simulink model "eVTOL_PX4_2023b"  (R2024b)
settings: Solver=ode4  StartTime=0  StopTime=inf  FixedStep=0.01  RelTol=1e-3
values from neighbouring files (symbols this model uses):
  aDl =     [initdata.mat]
  aDr =     [initdata.mat]
  aDyn =     [initdata.mat]
  Airport = init_airport('PHNL')    [initdata_HIL_eVTOL.m]
  aLat =     [initdata.mat]
  aLon =     [initdata.mat]
  D = Prop.D    [EOM_dt_MC.m]    (also in EOM_get_alf_dt_de_prop_evtol.m = CD * QS)
  dt0 = X(2)    [EOM_get_alf_dt_de_prop_evtol.m]    (also in initdata.mat = 0.258252593971; initdata_HIL_eVTOL.m = EOM_dt_MC)
  EAS0 = TAS0 / EAS2TAS    [initdata_HIL_eVTOL.m]
  FCS = init_FCS    [initdata_HIL_eVTOL.m]
  General = init_layoutdata    [EOM_dt_MC.m]    (also in build_optimized_CA.m; initdata.mat = ; initdata_HIL_eVTOL.m)
  h0 = Con(1)    [EOM_get_alf_dt_de_prop_evtol.m]    (also in initdata.mat = 450; initdata_HIL_eVTOL.m = 50)
  mass = Con(3)    [EOM_get_alf_dt_de_prop_evtol.m]    (also in initdata.mat = 2255.54; initdata_HIL_eVTOL.m = 7)
  Motor = init_motor_evtol    [EOM_dt_MC.m]    (also in initdata.mat = []; initdata_HIL_eVTOL.m)
  Prop = init_propeller_evtol_new    [EOM_dt_MC.m]    (also in initdata_HIL_eVTOL.m)
  R2D = 180/pi    (= 57.2957795131)    [EOM_get_alf_dt_de_prop_evtol.m]    (also in init_FCS.m; init_aerodata_evtol.m; init_airport.m; initdata.mat)
  SAMPLE_TIME = 0.01    [initdata_HIL_eVTOL.m]
  theta0 = -0.0510981441662    [initdata.mat]
undefined symbols (not defined in the file or in its folder): A1, aDa, aDe, aero, asbhl20env, B1, C1, de0, Earth, Environment, INIT_Data, InitData, Kd, Kp, magnitude, Newton, pProp, Raphson, Tc, WGS84
libraries: simulink_extras x63, vrlib x48, sharedtransform x28, simulink x22, slpidlib x20, sharedutil x20, matrix_library x18, aerolibwindfilters x12, aerolibobsolete x8, aerolibasang x8, aerolibatmos2 x6, aerolibfltsims x6
(part 1 of 17)
settings Model: SimulationMode=accelerator  Creator=Administrator  LastModifiedBy=ZDB
settings SolverCC: EnableFixedStepZeroCrossing=on
settings OptimizationCC: ReuseModelBlockBuffer=off
settings DebuggingCC: UnconnectedInputMsg=warning  UnconnectedOutputMsg=warning  UnconnectedLineMsg=warning
settings ModelReferenceCC: EnableRefExpFcnMdlSchedulingChecks=on
settings RTWCC: GPUComputeCapability=3.5  DLArmComputeVersion=19.05

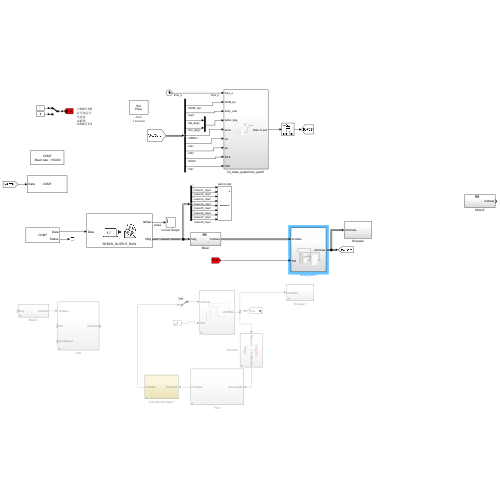
[thumbnail: Simulink's stored preview of the top-level diagram]
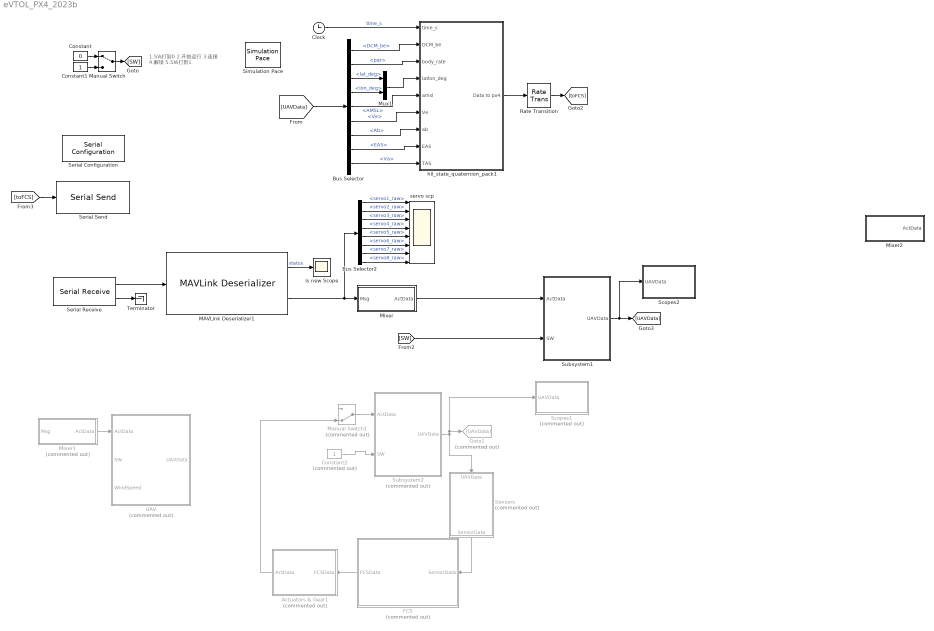
== system eVTOL_PX4_2023b ==
  note: 1.SW打到0
      | 2.开始运行
      | 3.连接
      | 4.解锁
      | 5.SW打到1
  Actuators & Gear1 : Subsystem  Commented=on
  Bus Selector : BusSelector  OutputSignals=DCM_be,pqr,lat_deg,lon_deg,AMSL,Ve,Ab,EAS,Va
  Bus Selector2 : BusSelector  OutputSignals=Payload.servo1_raw,Payload.servo2_raw,Payload.servo3_raw,Payload.servo4_raw,Payload.servo5_raw,Payload.servo6_raw,Payload.servo7_raw,Payload.servo8_raw
  Clock : Clock
  Constant : Constant  Value=0
  Constant1 : Constant
  Constant2 : Constant  Commented=on
  FCS : Subsystem  Commented=on
  Goto1 : Goto  Commented=on  GotoTag=UAVData
  MAVLink Deserializer1 : uavmavlinklib/MAVLink Deserializer  dialectSource=Select from standard MAVLink dialects  dialect=common.xml  dialectCustom=common.xml  version=2  messageType=SERVO_OUTPUT_RAW  inputDataLength=off  SystemIDFilter=off  systemID=1  ComponentIDFilter=off  componentID=1  queueMsg=off  queueMsgSize=50  dropNum=off
  Manual Switch : ManualSwitch
  Manual Switch1 : ManualSwitch  Commented=on  CurrentSetting=0
  Mixer : Subsystem
  Mixer1 : Subsystem  Commented=on
  Mixer2 : Subsystem
  Mux1 : Mux  Inputs=2
  Rate Transition : RateTransition  OutPortSampleTime=0.01
  Scopes1 : Subsystem  Commented=on
  Scopes2 : Subsystem
  Sensors : Subsystem  Commented=on
  Serial Configuration : instrumentseriallib/Serial Configuration  Priority=-200000  PortSel=COM7  Port=COM7  ComPort=COM7  BaudRate=115200  DataBits=8  Parity=none  StopBits=1  ByteOrder=little-endian  FlowControl=none  Timeout=10  SimulateUsing=Interpreted execution  BlockInModel=on  aMode=1
  Serial Receive : instrumentseriallib/Serial Receive  PortSel=COM7  Port=COM7  ComPort=COM7  DataType=uint8  SaveDataType=uint8  ToggleHeader=off  Header=[253 37]  ToggleDataSize=on  DataSize=[49]  ToggleTerminator=off  Terminator=<none>  CustomTerminator=[]  InputFormat=Column major  EnableBlockingMode=off  ActionDataUnavailable=Output last received value  ActionWhenDataUnavailable=Output last received value  CustomValue=0  SampleTime=SAMPLE_TIME  SimulateUsing=Interpreted execution  BlockInModel=on  aMode=1
  Serial Send : instrumentseriallib/Serial Send  Priority=1  PortSel=COM7  Port=COM7  ComPort=COM7  Header=[]  Terminator=<none>  CustomTerminator=[]  EnableBlockingMode=off  SimulateUsing=Interpreted execution  BlockInModel=on  aMode=1
  Simulation Pace : aerolibanimutils/Simulation Pace  SimulationPace=1  SleepMode=Auto  OutputPaceError=off  SampleTime=-1
  Subsystem1 : Subsystem
  Subsystem2 : Subsystem  Commented=on
  Terminator : Terminator
  UAV : Subsystem  Commented=on
  hil_state_quaternion_pack1 : Subsystem
  is new Scope : Scope
  servo scp : Scope  NumInputPorts=8
  wires:
  Actuators & Gear1/1(ActData) -> Manual Switch1/2
  FCS/1(FCSData) -> Actuators & Gear1/1(FCSData)
  Sensors/1(SensorData) -> FCS/1(SensorData)
  Manual Switch/1 -> [SW]
  Bus Selector/5 -> hil_state_quaternion_pack1/5(amsl)  "<AMSL>"
  Bus Selector/4 -> Mux1/2  "<lon_deg>"
  [toFCS] -> Serial Send/1
  Bus Selector/9 -> hil_state_quaternion_pack1/9(TAS)  "<Va>"
  Bus Selector/6 -> hil_state_quaternion_pack1/6(Ve)  "<Ve>"
  Constant1/1 -> Manual Switch/2
  Serial Receive/1 -> MAVLink Deserializer1/1
  MAVLink Deserializer1/1 -> is new Scope/1  "status"
  Constant/1 -> Manual Switch/1
  Bus Selector/8 -> hil_state_quaternion_pack1/8(EAS)  "<EAS>"
  Constant2/1 -> Subsystem2/2(SW)
  Bus Selector/3 -> Mux1/1  "<lat_deg>"
  Bus Selector/1 -> hil_state_quaternion_pack1/2(DCM_be)  "<DCM_be>"
  hil_state_quaternion_pack1/1(Data to px4) -> Rate Transition/1
  Rate Transition/1 -> [toFCS]
  Bus Selector/7 -> hil_state_quaternion_pack1/7(ab)  "<Ab>"
  Mux1/1 -> hil_state_quaternion_pack1/4(latlon_deg)
  Bus Selector/2 -> hil_state_quaternion_pack1/3(body_rate)  "<pqr>"
  [UAVData] -> Bus Selector/1
  Clock/1 -> hil_state_quaternion_pack1/1(time_s)  "time_s"
  Serial Receive/2 -> Terminator/1
  Subsystem2/1(UAVData) -> Goto1/1, Scopes1/1(UAVData), Sensors/1(UAVData)
  Mixer1/1(ActData) -> UAV/1(ActData)
  Manual Switch1/1 -> Subsystem2/1(ActData)
  [SW] -> Subsystem1/2(SW)
  Subsystem1/1(UAVData) -> [UAVData], Scopes2/1(UAVData)
  Bus Selector2/6 -> servo scp/6  "<servo6_raw>"
  Bus Selector2/3 -> servo scp/3  "<servo3_raw>"
  Bus Selector2/4 -> servo scp/4  "<servo4_raw>"
  Bus Selector2/5 -> servo scp/5  "<servo5_raw>"
  MAVLink Deserializer1/2 -> Bus Selector2/1, Mixer/1(Msg)
  Bus Selector2/1 -> servo scp/1  "<servo1_raw>"
  Bus Selector2/2 -> servo scp/2  "<servo2_raw>"
  Bus Selector2/7 -> servo scp/7  "<servo7_raw>"
  Bus Selector2/8 -> servo scp/8  "<servo8_raw>"
  Mixer/1(ActData) -> Subsystem1/1(ActData)

== system eVTOL_PX4_2023b/Actuators & Gear1 ==
  FCSData : Inport
  1-D Lookup Table1 : Lookup_n-D  NumberOfTableDimensions=1  BreakpointsForDimension1=[0, 0.8,1.2,1.57]  Table=[72.43*pi/180,60/57.3,40/57.3, 13*pi/180]  InternalRulePriority=Speed  RndMeth=Simplest
  Bus Creator : BusCreator  Inputs=3
  Bus Creator1 : BusCreator  Inputs=8
  Bus Creator2 : BusCreator  Inputs=2
  Bus Selector : BusSelector  OutputSignals=ACTCMD.dl_cmd,ACTCMD.dt_final,ACTCMD.dr_cmd,ACTCMD.da_cmd,SensorData.Va,FCSCMD.icmd
  Demux : Demux  Outputs=6
  Gain{2,4..11} (9 alike) : Gain
  Max : MinMax  Function=max  Inputs=2
  Mux1 : Mux
  Mux2 : Mux
  Radians to Degrees1 : simulink_extras/Transformations/Radians to Degrees
  Radians to Degrees2 : simulink_extras/Transformations/Radians to Degrees
  Radians to Degrees3 : simulink_extras/Transformations/Radians to Degrees
  Rate Limiter : RateLimiter  FallingSlewLimit=-0.2  SampleTimeMode=inherited
  Saturation1 : Saturate  UpperLimit=25/57.3  LowerLimit=-25/57.3
  Saturation3 : Saturate  UpperLimit=25/57.3  LowerLimit=-25/57.3
  Scope1 : Scope
  Scope2 : Scope
  "[-25,25]" : Saturate  UpperLimit=25/57.3  LowerLimit=-25/57.3
  control output FW : Scope  NumInputPorts=3
  safe i_min : Lookup_n-D  NumberOfTableDimensions=1  BreakpointsForDimension1=[0, 5, 10, 15, 22, 30, 38, 46, 54, 60, 63, 65,80]  Table=[1.22,1.19,1.13,1.05,0.96,0.84,0.7,0.52,0.31,0.14,0.04,0,0]  InternalRulePriority=Speed  RndMeth=Simplest
  ActData : Outport  VectorParamsAs1DForOutWhenUnconnected=off
  tag scope: i=global, theta__b=global
  wires:
  Bus Creator/1 -> Bus Creator2/1  "Act_surface"
  "[-25,25]"/1 -> Radians to Degrees1/1, Bus Creator/2  "dr"
  Saturation3/1 -> Bus Creator/3, Radians to Degrees2/1  "da"
  Saturation1/1 -> Radians to Degrees3/1, Bus Creator/1  "dl"
  Radians to Degrees3/1 -> control output FW/1  "da"
  Radians to Degrees1/1 -> control output FW/2  "de"
  Radians to Degrees2/1 -> control output FW/3  "dr"
  Gain4/1 -> "[-25,25]"/1
  Gain5/1 -> Saturation3/1
  Bus Creator1/1 -> Bus Creator2/2  "Act_T"
  Gain6/1 -> Saturation1/1  "dl"
  FCSData/1 -> Bus Selector/1
  Bus Selector/1 -> Gain6/1  "<dl_cmd>"
  Gain2/1 -> Bus Creator1/1  "dt_1"
  Gain7/1 -> Bus Creator1/2  "dt_2"
  Gain8/1 -> Bus Creator1/3  "dt_3"
  Gain9/1 -> Bus Creator1/4  "dt_4"
  Gain10/1 -> Bus Creator1/5  "dt_5"
  Gain11/1 -> Bus Creator1/6  "dt_6"
  Bus Selector/5 -> safe i_min/1  "<Va>"
  safe i_min/1 -> Max/2
  Max/1 -> Rate Limiter/1  "i"
  1-D Lookup Table1/1 -> [theta__b], Scope2/1  "theta_b"
  Bus Selector/6 -> Max/1  "<icmd>"
  Demux/1 -> Gain2/1
  Demux/2 -> Gain7/1
  Demux/3 -> Gain8/1
  Demux/4 -> Gain9/1
  Demux/5 -> Gain10/1
  Demux/6 -> Gain11/1
  Bus Selector/2 -> Demux/1  "<dt_final>"
  Rate Limiter/1 -> 1-D Lookup Table1/1, Scope1/1, [i]  "i"
  Bus Selector/3 -> Gain4/1  "<dr_cmd>"
  Bus Selector/4 -> Gain5/1  "<da_cmd>"
  Bus Creator2/1 -> ActData/1
  [i] -> Mux1/1  "tilt16"
  [theta__b] -> Mux2/4  "theta_b4"
  [theta__b] -> Mux2/1  "theta_b16"
  [theta__b] -> Mux2/3  "theta_b3"
  [i] -> Mux1/3  "tilt2"
  Mux1/1 -> Bus Creator1/7  "i"
  [i] -> Mux1/4  "tilt5"
  [theta__b] -> Mux2/2  "theta_b25"
  Mux2/1 -> Bus Creator1/8  "theta_b"
  [i] -> Mux1/2  "tilt34"

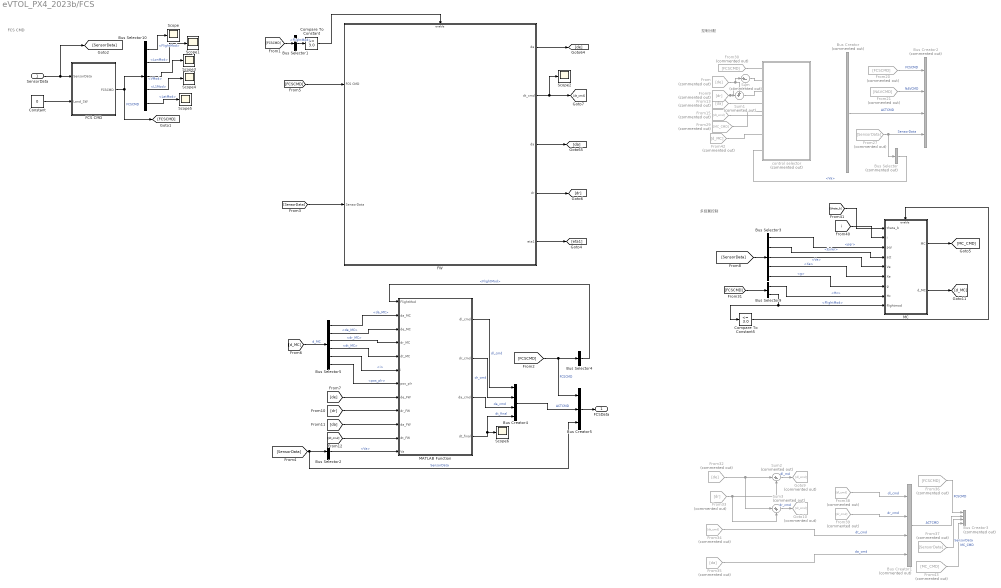
== system eVTOL_PX4_2023b/FCS ==
  note: 控制分配
  note: 多旋翼控制
  note: FCS CMD
  SensorData : Inport
  Bus Creator{,1..3} (4 alike) : BusCreator  Commented=on  Inputs=4
  Bus Creator4 : BusCreator  Inputs=4
  Bus Creator5 : BusCreator  Inputs=3
  Bus Selector : BusSelector  Commented=on  OutputSignals=Va
  Bus Selector1 : BusSelector  OutputSignals=FlightMod
  Bus Selector10 : BusSelector  OutputSignals=FlightMod,LonMod,VMod,L1Mod,LatMod
  Bus Selector2 : BusSelector  OutputSignals=Va
  Bus Selector3 : BusSelector  OutputSignals=pqr,Euler,Ve,Xe,g
  Bus Selector4 : BusSelector  OutputSignals=FlightMod
  Bus Selector5 : BusSelector  OutputSignals=da_MC,de_MC,dr_MC,dt_MC,i,pos_plr
  Bus Selector9 : BusSelector  OutputSignals=Hc,FlightMod
  Compare To Constant : simulink/Logic and Bit Operations/Compare To Constant  relop=>=  const=3.0  OutDataTypeStr=boolean
  Compare To Constant5 : simulink/Logic and Bit Operations/Compare To Constant  relop=<=  const=3.0  OutDataTypeStr=boolean
  Constant : Constant  Value=0
  FCS CMD : Subsystem
  FW : Subsystem
  From : From  Commented=on  GotoTag=de
  From13 : From  Commented=on  GotoTag=da
  From15 : From  Commented=on  GotoTag=dt_cmd
  From20 : From  Commented=on  GotoTag=FCSCMD
      settings: CloseFcn=tagdialog Close
  From21 : From  Commented=on  GotoTag=NAVCMD
      settings: CloseFcn=tagdialog Close
  From27 : From  Commented=on  GotoTag=SensorData
  From29 : From  Commented=on  GotoTag=MC_CMD
  From30 : From  Commented=on  GotoTag=FCSCMD
      settings: CloseFcn=tagdialog Close
  From32 : From  Commented=on  GotoTag=de
  From33 : From  Commented=on  GotoTag=dr
  From34 : From  Commented=on  GotoTag=dt_cmd
  From35 : From  Commented=on  GotoTag=da
  From36 : From  Commented=on  GotoTag=FCSCMD
  From37 : From  Commented=on  GotoTag=SensorData
  From38 : From  Commented=on  GotoTag=dl_cmd
  From39 : From  Commented=on  GotoTag=dr_cmd
  From42 : From  Commented=on  GotoTag=d_MC
  From43 : From  Commented=on  GotoTag=MC_CMD
  From9 : From  Commented=on  GotoTag=dr
  Goto10 : Goto  Commented=on  GotoTag=dr_cmd
  Goto9 : Goto  Commented=on  GotoTag=dl_cmd
  MATLAB Function : MATLAB Function  TreatAsAtomicUnit=on
  MC : Subsystem
  Scope{,1..6} (7 alike) : Scope
  Sum : Sum  Commented=on  Inputs=|+-
  Sum1 : Sum  Commented=on  Inputs=++|
  Sum2 : Sum  Commented=on  Inputs=|+-
  Sum3 : Sum  Commented=on  Inputs=|++
  control selector : Subsystem  Commented=on
  FCSData : Outport  VectorParamsAs1DForOutWhenUnconnected=off
  wires:
  Bus Creator/1 -> Bus Creator2/3  "ACTCMD"
  SensorData/1 -> FCS CMD/1(SensorData), [SensorData]
  FCS CMD/1(FCSCMD) -> Bus Selector10/1, [FCSCMD]  "FCSCMD"
  From20/1 -> Bus Creator2/1  "FCSCMD"
  From21/1 -> Bus Creator2/2  "NAVCMD"
  From30/1 -> ?
  [SensorData] -> Bus Selector3/1
  Bus Selector3/1 -> MC/3(pqr)  "<pqr>"
  Bus Selector3/2 -> MC/4(att)  "<Euler>"
  Bus Selector3/3 -> MC/5(Ve)  "<Ve>"
  Bus Selector3/4 -> MC/6(Xe)  "<Xe>"
  Constant/1 -> FCS CMD/2(Land_SW)
  Bus Selector3/5 -> MC/7(g)  "<g>"
  From/1 -> Sum1/1, Sum/1
  From9/1 -> Sum/2, Sum1/2
  Sum/1 -> ?
  Sum1/1 -> ?
  From13/1 -> ?
  From15/1 -> ?
  From27/1 -> Bus Selector/1, Bus Creator2/4  "SensorData"
  From29/1 -> ?
  Bus Selector/1 -> ?  "<Va>"
  [FCSCMD] -> Bus Selector9/1
  Bus Selector9/1 -> MC/8(Hc)  "<Hc>"
  Bus Selector10/1 -> Scope/1  "<FlightMod>"
  Bus Selector10/2 -> Scope1/1  "<LonMod>"
  Bus Selector10/3 -> Scope3/1  "<VMod>"
  Bus Selector10/4 -> Scope4/1  "<L1Mod>"
  Bus Selector10/5 -> Scope5/1  "<LatMod>"
  From33/1 -> Sum3/2, Sum2/2
  From32/1 -> Sum3/1, Sum2/1
  From34/1 -> Bus Creator1/3  "dt_cmd"
  From35/1 -> Bus Creator1/4  "da_cmd"
  Bus Creator1/1 -> Bus Creator3/2  "ACTCMD"
  From36/1 -> Bus Creator3/1  "FCSCMD"
  From37/1 -> Bus Creator3/3  "SensorData"
  Sum2/1 -> Goto9/1  "dl_md"
  Sum3/1 -> Goto10/1  "dr_cmd"
  From39/1 -> Bus Creator1/2  "dr_cmd"
  From38/1 -> Bus Creator1/1  "dl_cmd"
  Bus Selector9/2 -> Compare To Constant5/1, MC/9(flightmod)  "<FlightMod>"
  [i] -> MC/2(i)
  [theta_b] -> MC/1(theta_b)
  From42/1 -> ?
  ? -> Bus Creator/1  "dl_cmd"
  ? -> Bus Creator/2  "dr_cmd"
  ? -> Bus Creator/3  "da_cmd"
  ? -> Bus Creator/4  "dt_cmd"
  From43/1 -> Bus Creator3/4  "MC_CMD"
  FW/1(de) -> [de]
  [FCSCMD] -> FW/1(FCS CMD)
  [SensorData] -> FW/2(SensorData)
  FW/5(eta1) -> [eta1]
  FW/4(dr) -> [dr]
  FW/3(da) -> [da]
  FW/2(dt_cmd) -> Scope2/1, [dt_cmd]
  [FCSCMD] -> Bus Selector1/1
  Bus Selector1/1 -> Compare To Constant/1  "<FlightMod>"
  Compare To Constant/1 -> FW/Enable
  MATLAB Function/1(dl_cmd) -> Bus Creator4/1  "dl_cmd"
  MATLAB Function/2(dr_cmd) -> Bus Creator4/2  "dr_cmd"
  MATLAB Function/3(da_cmd) -> Bus Creator4/3  "da_cmd"
  MATLAB Function/4(dt_final) -> Scope6/1, Bus Creator4/4  "dt_final"
  Bus Creator4/1 -> Bus Creator5/2  "ACTCMD"
  [SensorData] -> Bus Creator5/3, Bus Selector2/1  "SensorData"
  Bus Selector2/1 -> MATLAB Function/12(Va)  "<Va>"
  [FCSCMD] -> Bus Selector4/1, Bus Creator5/1  "FCSCMD"
  Bus Creator5/1 -> FCSData/1
  Bus Selector4/1 -> MATLAB Function/1(FlightMod)  "<FlightMod>"
  [d_MC] -> Bus Selector5/1  "d_MC"
  Bus Selector5/6 -> MATLAB Function/7(pos_plr)  "<pos_plr>"
  Bus Selector5/1 -> MATLAB Function/2(da_MC)  "<da_MC>"
  Bus Selector5/2 -> MATLAB Function/3(de_MC)  "<de_MC>"
  Bus Selector5/3 -> MATLAB Function/4(dr_MC)  "<dr_MC>"
  Bus Selector5/4 -> MATLAB Function/5(dt_MC)  "<dt_MC>"
  Bus Selector5/5 -> MATLAB Function/6(i)  "<i>"
  [de] -> MATLAB Function/8(de_FW)
  [dr] -> MATLAB Function/9(dr_FW)
  [da] -> MATLAB Function/10(da_FW)
  [dt_cmd] -> MATLAB Function/11(dt_FW)
  MC/1(MC) -> [MC_CMD]
  MC/2(d_MC) -> [d_MC]
  Compare To Constant5/1 -> MC/Enable

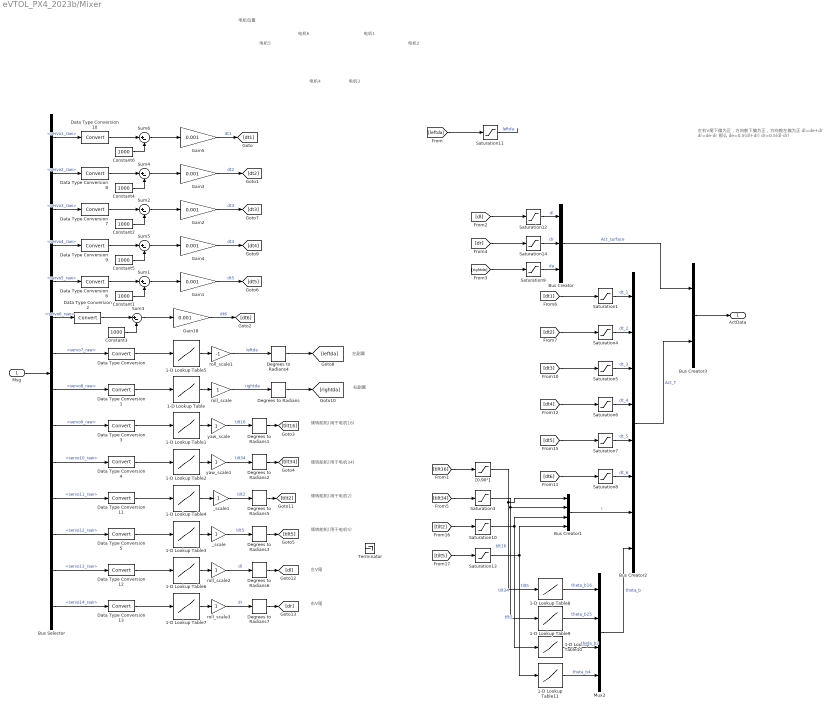
== system eVTOL_PX4_2023b/Mixer ==
  note: 电机1
  note: 电机位置
  note: 左副翼
  note: 左右V尾下偏为正，方向舵下偏为正，方向舵左偏为正
      | dl=de+dr
      | dr=de-dr
      | 那么
      | de=0.5(dl+dr)
      | dr=0.5(dl-dr)
  note: 右副翼
  note: 倾转舵机(用于电机16)
  note: 左V尾
  note: 右V尾
  note: 倾转舵机(用于电机34)
  note: 倾转舵机(用于电机2)
  note: 倾转舵机(用于电机5)
  note: 电机2
  note: 电机3
  note: 电机4
  note: 电机5
  note: 电机6
  Msg : Inport
  1-D Lookup Table{,5..7} (4 alike) : Lookup_n-D  NumberOfTableDimensions=1  BreakpointsForDimension1=[1000, 1500, 2000]  Table=[-30, 0, 30]  InternalRulePriority=Speed  RndMeth=Simplest
  1-D Lookup Table{1..4} (4 alike) : Lookup_n-D  NumberOfTableDimensions=1  BreakpointsForDimension1=[1000, 1500, 2000]  Table=[90, 45, 0]  InternalRulePriority=Speed  RndMeth=Simplest
  1-D Lookup Table{8..11} (4 alike) : Lookup_n-D  NumberOfTableDimensions=1  BreakpointsForDimension1=[0, 0.8,1.2,1.57]  Table=[72.43*pi/180,60/57.3,40/57.3, 13*pi/180]  InternalRulePriority=Speed  RndMeth=Simplest
  Bus Creator : BusCreator  Inputs=3
  Bus Creator1 : BusCreator  Inputs=4
  Bus Creator2 : BusCreator  Inputs=8
  Bus Creator3 : BusCreator  Inputs=2
  Bus Selector : BusSelector  OutputSignals=Payload.servo1_raw,Payload.servo2_raw,Payload.servo3_raw,Payload.servo4_raw,Payload.servo5_raw,Payload.servo6_raw,Payload.servo7_raw,Payload.servo8_raw,Payload.servo9_raw,Payload.servo10_raw,Payload.servo11_raw,Payload.servo12_raw,Payload.servo13_raw,Payload.servo14_raw
  Constant{1..6} (6 alike) : Constant  Value=1000
  Data Type Conversion{,1..13} (14 alike) : DataTypeConversion  SaturateOnIntegerOverflow=off  RndMeth=Floor
  Degrees to Radians{,1..7} (8 alike) : simulink_extras/Transformations/Degrees to Radians
  Gain{1..5,18} (6 alike) : Gain  Gain=0.001
  Mux2 : Mux
  Saturation{1,4..8} (6 alike) : Saturate  UpperLimit=1  LowerLimit=0
  Saturation10 : Saturate  UpperLimit=90/57.3  LowerLimit=0
  Saturation{9,11..12,14} (4 alike) : Saturate  UpperLimit=25/57.3  LowerLimit=-25/57.3
  Saturation13 : Saturate  UpperLimit=90/57.3  LowerLimit=0
  Saturation3 : Saturate  UpperLimit=90/57.3  LowerLimit=0
  Sum{1..6} (6 alike) : Sum  Inputs=|+-
  Terminator : Terminator
  "[0,90°]" : Saturate  UpperLimit=90/57.3  LowerLimit=0
  _scale : Gain
  _scale1 : Gain
  roll_scale : Gain
  roll_scale1 : Gain  Gain=-1
  roll_scale2 : Gain
  roll_scale3 : Gain
  yaw_scale : Gain
  yaw_scale1 : Gain
  ActData : Outport  VectorParamsAs1DForOutWhenUnconnected=off
  wires:
  Bus Selector/6 -> Data Type Conversion2/1  "<servo6_raw>"
  Bus Selector/7 -> Data Type Conversion/1  "<servo7_raw>"
  Bus Selector/8 -> Data Type Conversion1/1  "<servo8_raw>"
  Constant3/1 -> Sum3/2
  Sum3/1 -> Gain18/1
  Degrees to Radians4/1 -> [leftda]
  Degrees to Radians/1 -> [rightda]
  1-D Lookup Table1/1 -> yaw_scale/1
  [leftda] -> Saturation11/1
  Saturation11/1 -> ?  "leftda"
  [dl] -> Saturation12/1
  Saturation12/1 -> Bus Creator/1  "dl"
  "[0,90°]"/1 -> 1-D Lookup Table8/1, Bus Creator1/1  "tilt16"
  Saturation3/1 -> 1-D Lookup Table9/1, Bus Creator1/2  "tilt34"
  1-D Lookup Table3/1 -> _scale/1
  1-D Lookup Table2/1 -> yaw_scale1/1
  Gain18/1 -> [dt6]  "dt6"
  Bus Selector/9 -> Data Type Conversion3/1  "<servo9_raw>"
  Bus Selector/10 -> Data Type Conversion4/1  "<servo10_raw>"
  Degrees to Radians1/1 -> [tilt16]
  Degrees to Radians2/1 -> [tilt34]
  Degrees to Radians3/1 -> [tilt5]
  _scale/1 -> Degrees to Radians3/1  "tilt5"
  yaw_scale/1 -> Degrees to Radians1/1  "tilt16"
  yaw_scale1/1 -> Degrees to Radians2/1  "tilt34"
  Data Type Conversion/1 -> 1-D Lookup Table5/1
  Data Type Conversion1/1 -> 1-D Lookup Table/1
  Data Type Conversion3/1 -> 1-D Lookup Table1/1
  Data Type Conversion4/1 -> 1-D Lookup Table2/1
  Data Type Conversion5/1 -> 1-D Lookup Table3/1
  roll_scale/1 -> Degrees to Radians/1  "rightda"
  1-D Lookup Table/1 -> roll_scale/1
  [dr] -> Saturation14/1
  [tilt16] -> "[0,90°]"/1
  [tilt34] -> Saturation3/1
  1-D Lookup Table5/1 -> roll_scale1/1
  roll_scale1/1 -> Degrees to Radians4/1  "leftda"
  Data Type Conversion2/1 -> Sum3/1
  Bus Selector/5 -> Data Type Conversion6/1  "<servo5_raw>"
  Constant1/1 -> Sum1/2
  Data Type Conversion6/1 -> Sum1/1
  Sum1/1 -> Gain1/1
  Gain1/1 -> [dt5]  "dt5"
  Bus Selector/4 -> Data Type Conversion9/1  "<servo4_raw>"
  Constant5/1 -> Sum5/2
  Data Type Conversion9/1 -> Sum5/1
  Sum5/1 -> Gain4/1
  Gain4/1 -> [dt4]  "dt4"
  Bus Selector/3 -> Data Type Conversion7/1  "<servo3_raw>"
  Constant2/1 -> Sum2/2
  Data Type Conversion7/1 -> Sum2/1
  Sum2/1 -> Gain2/1
  Gain2/1 -> [dt3]  "dt3"
  Bus Selector/2 -> Data Type Conversion8/1  "<servo2_raw>"
  Constant4/1 -> Sum4/2
  Data Type Conversion8/1 -> Sum4/1
  Sum4/1 -> Gain3/1
  Gain3/1 -> [dt2]  "dt2"
  Bus Selector/1 -> Data Type Conversion10/1  "<servo1_raw>"
  Constant6/1 -> Sum6/2
  Data Type Conversion10/1 -> Sum6/1
  Sum6/1 -> Gain5/1
  Gain5/1 -> [dt1]  "dt1"
  Data Type Conversion11/1 -> 1-D Lookup Table4/1
  Degrees to Radians5/1 -> [tilt2]
  _scale1/1 -> Degrees to Radians5/1  "tilt2"
  Bus Selector/11 -> Data Type Conversion11/1  "<servo11_raw>"
  1-D Lookup Table4/1 -> _scale1/1
  Data Type Conversion12/1 -> 1-D Lookup Table6/1
  Degrees to Radians6/1 -> [dl]
  roll_scale2/1 -> Degrees to Radians6/1  "dl"
  Bus Selector/13 -> Data Type Conversion12/1  "<servo13_raw>"
  1-D Lookup Table6/1 -> roll_scale2/1
  Data Type Conversion13/1 -> 1-D Lookup Table7/1
  Degrees to Radians7/1 -> [dr]
  roll_scale3/1 -> Degrees to Radians7/1  "dr"
  Bus Selector/14 -> Data Type Conversion13/1  "<servo14_raw>"
  1-D Lookup Table7/1 -> roll_scale3/1
  Bus Selector/12 -> Data Type Conversion5/1  "<servo12_raw>"
  [dt1] -> Saturation1/1
  Saturation1/1 -> Bus Creator2/1  "dt_1"
  [dt2] -> Saturation4/1
  Saturation4/1 -> Bus Creator2/2  "dt_2"
  [dt3] -> Saturation5/1
  Saturation5/1 -> Bus Creator2/3  "dt_3"
  Saturation7/1 -> Bus Creator2/5  "dt_5"
  Saturation6/1 -> Bus Creator2/4  "dt_4"
  [dt4] -> Saturation6/1
  [dt6] -> Saturation8/1
  Saturation8/1 -> Bus Creator2/6  "dt_6"
  [dt5] -> Saturation7/1
  [rightda] -> Saturation9/1
  Saturation9/1 -> Bus Creator/3  "da"
  [tilt2] -> Saturation10/1
  Saturation10/1 -> Bus Creator1/3, 1-D Lookup Table10/1  "tilt2"
  [tilt5] -> Saturation13/1
  Saturation13/1 -> Bus Creator1/4, 1-D Lookup Table11/1  "tilt5"
  Bus Creator3/1 -> ActData/1
  Bus Creator2/1 -> Bus Creator3/2  "Act_T"
  Bus Creator/1 -> Bus Creator3/1  "Act_surface"
  Saturation14/1 -> Bus Creator/2  "dr"
  Bus Creator1/1 -> Bus Creator2/7  "i"
  1-D Lookup Table8/1 -> Mux2/1  "theta_b16"
  1-D Lookup Table9/1 -> Mux2/2  "theta_b25"
  1-D Lookup Table10/1 -> Mux2/3  "theta_b3"
  1-D Lookup Table11/1 -> Mux2/4  "theta_b4"
  Mux2/1 -> Bus Creator2/8  "theta_b"
  Msg/1 -> Bus Selector/1
  ? -> ?  "y轴"
  ? -> ?  "x轴"

== system eVTOL_PX4_2023b/Mixer1 ==
  Msg : Inport
  1-D Lookup Table{,1..3,5} (5 alike) : Lookup_n-D  NumberOfTableDimensions=1  BreakpointsForDimension1=[1000, 1500, 2000]  Table=[-20, 0, 20]  InternalRulePriority=Speed  RndMeth=Simplest
  Bus Creator1 : BusCreator  Inputs=6
  Bus Selector : BusSelector  OutputSignals=Payload.servo1_raw,Payload.servo2_raw,Payload.servo3_raw,Payload.servo4_raw,Payload.servo5_raw,Payload.servo6_raw
  Constant3 : Constant  Value=1000
  Data Type Conversion{,1..5} (6 alike) : DataTypeConversion  SaturateOnIntegerOverflow=off  RndMeth=Floor
  Degrees to Radians{,1..4} (5 alike) : simulink_extras/Transformations/Degrees to Radians
  Gain18 : Gain  Gain=0.001
  Radians to Degrees : simulink_extras/Transformations/Radians to Degrees
  Radians to Degrees4 : simulink_extras/Transformations/Radians to Degrees
  Radians to Degrees5 : simulink_extras/Transformations/Radians to Degrees
  Saturation11 : Saturate  UpperLimit=1  LowerLimit=-1
  Saturation12 : Saturate  UpperLimit=1  LowerLimit=-1
  Saturation13 : Saturate  UpperLimit=1  LowerLimit=0
  Saturation14 : Saturate  UpperLimit=25/57.3  LowerLimit=-25/57.3
  Saturation2 : Saturate  UpperLimit=25/57.3  LowerLimit=-25/57.3
  Saturation3 : Saturate  UpperLimit=25/57.3  LowerLimit=-25/57.3
  Sum3 : Sum  Inputs=|+-
  da Scope : Scope
  de Scope : Scope
  dr Scope : Scope
  dt Scope : Scope
  pitch_scale : Gain  Gain=-1
  pitch_scale1 : Gain  Gain=-1
  roll_scale : Gain
  yaw_scale : Gain  Gain=-1
  yaw_scale1 : Gain
  ActData : Outport
  wires:
  Data Type Conversion2/1 -> Sum3/1
  pitch_scale1/1 -> Degrees to Radians4/1
  1-D Lookup Table5/1 -> pitch_scale1/1
  [dt6] -> Saturation3/1
  [dt5] -> Saturation2/1
  [dt4] -> Saturation14/1
  1-D Lookup Table/1 -> pitch_scale/1
  pitch_scale/1 -> Degrees to Radians/1
  Data Type Conversion5/1 -> 1-D Lookup Table3/1
  Data Type Conversion4/1 -> 1-D Lookup Table2/1
  Data Type Conversion3/1 -> 1-D Lookup Table1/1
  Data Type Conversion1/1 -> 1-D Lookup Table/1
  Data Type Conversion/1 -> 1-D Lookup Table5/1
  yaw_scale1/1 -> Degrees to Radians2/1
  yaw_scale/1 -> Degrees to Radians1/1
  roll_scale/1 -> Degrees to Radians3/1
  Radians to Degrees5/1 -> da Scope/1  "da"
  [dt1] -> Radians to Degrees5/1
  [dt4] -> Radians to Degrees4/1
  Radians to Degrees4/1 -> dr Scope/1  "dr"
  Degrees to Radians3/1 -> [dt6]
  Degrees to Radians2/1 -> [dt5]
  Degrees to Radians1/1 -> [dt4]
  Bus Selector/6 -> Data Type Conversion5/1  "<servo6_raw>"
  Bus Selector/5 -> Data Type Conversion4/1  "<servo5_raw>"
  Bus Selector/4 -> Data Type Conversion3/1  "<servo4_raw>"
  [dt3] -> dt Scope/1  "throttle"
  Radians to Degrees/1 -> de Scope/1  "de"
  Gain18/1 -> [dt3]
  [dt2] -> Radians to Degrees/1
  1-D Lookup Table2/1 -> yaw_scale1/1
  1-D Lookup Table3/1 -> roll_scale/1
  Saturation3/1 -> Bus Creator1/6  "wheel"
  Saturation2/1 -> Bus Creator1/5  "flap"
  Saturation14/1 -> Bus Creator1/4  "dr"
  Saturation13/1 -> Bus Creator1/3  "dt"
  [dt3] -> Saturation13/1
  Saturation12/1 -> Bus Creator1/2  "de"
  [dt2] -> Saturation12/1
  Saturation11/1 -> Bus Creator1/1  "da"
  [dt1] -> Saturation11/1
  1-D Lookup Table1/1 -> yaw_scale/1
  Degrees to Radians/1 -> [dt2]  "dt1"
  Degrees to Radians4/1 -> [dt1]  "dt1"
  Bus Creator1/1 -> ActData/1
  Sum3/1 -> Gain18/1
  Constant3/1 -> Sum3/2
  Bus Selector/2 -> Data Type Conversion1/1  "<servo2_raw>"
  Bus Selector/1 -> Data Type Conversion/1  "<servo1_raw>"
  Bus Selector/3 -> Data Type Conversion2/1  "<servo3_raw>"
  Msg/1 -> Bus Selector/1

== system eVTOL_PX4_2023b/Mixer2 ==
  note: 电机1
  note: 电机位置
  note: 左右V尾下偏为正，方向舵下偏为正，方向舵左偏为正
      | dl=de+dr
      | dr=de-dr
      | 那么
      | de=0.5(dl+dr)
      | dr=0.5(dl-dr)
  note: 电机2
  note: 电机3
  note: 电机4
  note: 电机5
  note: 电机6
  0.63 : Step  Time=10  After=0.63  SampleTime=0
  0.67 : Step  Time=10  After=0.67  SampleTime=0
  0.7 : Step  Time=10  After=0.7  SampleTime=0
  1-D Lookup Table{8..11} (4 alike) : Lookup_n-D  NumberOfTableDimensions=1  BreakpointsForDimension1=[0, 0.8,1.2,1.57]  Table=[72.43*pi/180,60/57.3,40/57.3, 13*pi/180]  InternalRulePriority=Speed  RndMeth=Simplest
  Bus Creator : BusCreator  Inputs=3
  Bus Creator2 : BusCreator  Inputs=8
  Bus Creator3 : BusCreator  Inputs=2
  Constant13 : Constant  Value=0
  Constant7 : Constant  Value=1.57
  Mux1 : Mux
  Mux2 : Mux
  Saturation{1,4..8} (6 alike) : Saturate  UpperLimit=1  LowerLimit=0
  Saturation10 : Saturate  UpperLimit=90/57.3  LowerLimit=0
  Saturation12 : Saturate  UpperLimit=25/57.3  LowerLimit=-25/57.3
  Saturation13 : Saturate  UpperLimit=90/57.3  LowerLimit=0
  Saturation14 : Saturate  UpperLimit=25/57.3  LowerLimit=-25/57.3
  Saturation3 : Saturate  UpperLimit=90/57.3  LowerLimit=0
  Saturation9 : Saturate  UpperLimit=25/57.3  LowerLimit=-25/57.3
  "[0,90°]" : Saturate  UpperLimit=90/57.3  LowerLimit=0
  ActData : Outport  VectorParamsAs1DForOutWhenUnconnected=off
  wires:
  Saturation12/1 -> Bus Creator/1  "dl"
  "[0,90°]"/1 -> 1-D Lookup Table8/1, Mux1/1  "tilt16"
  Saturation3/1 -> 1-D Lookup Table9/1, Mux1/2  "tilt34"
  Constant7/1 -> Saturation10/1, Saturation3/1, "[0,90°]"/1, Saturation13/1
  Saturation1/1 -> Bus Creator2/1  "dt_1"
  Saturation4/1 -> Bus Creator2/2  "dt_2"
  Saturation5/1 -> Bus Creator2/3  "dt_3"
  Saturation7/1 -> Bus Creator2/5  "dt_5"
  Saturation6/1 -> Bus Creator2/4  "dt_4"
  Saturation8/1 -> Bus Creator2/6  "dt_6"
  Constant13/1 -> Saturation9/1, Saturation14/1, Saturation12/1
  Saturation9/1 -> Bus Creator/3  "da"
  Saturation10/1 -> 1-D Lookup Table10/1, Mux1/3  "tilt2"
  Saturation13/1 -> 1-D Lookup Table11/1, Mux1/4  "tilt5"
  Bus Creator3/1 -> ActData/1
  Bus Creator2/1 -> Bus Creator3/2  "Act_T"
  Bus Creator/1 -> Bus Creator3/1  "Act_surface"
  Saturation14/1 -> Bus Creator/2  "dr"
  Mux1/1 -> Bus Creator2/7  "i"
  1-D Lookup Table8/1 -> Mux2/1  "theta_b16"
  1-D Lookup Table9/1 -> Mux2/2  "theta_b25"
  1-D Lookup Table10/1 -> Mux2/3  "theta_b3"
  1-D Lookup Table11/1 -> Mux2/4  "theta_b4"
  Mux2/1 -> Bus Creator2/8  "theta_b"
  ? -> ?  "y轴"
  ? -> ?  "x轴"
  0.7/1 -> Saturation8/1, Saturation1/1
  0.67/1 -> Saturation7/1, Saturation4/1
  0.63/1 -> Saturation6/1, Saturation5/1

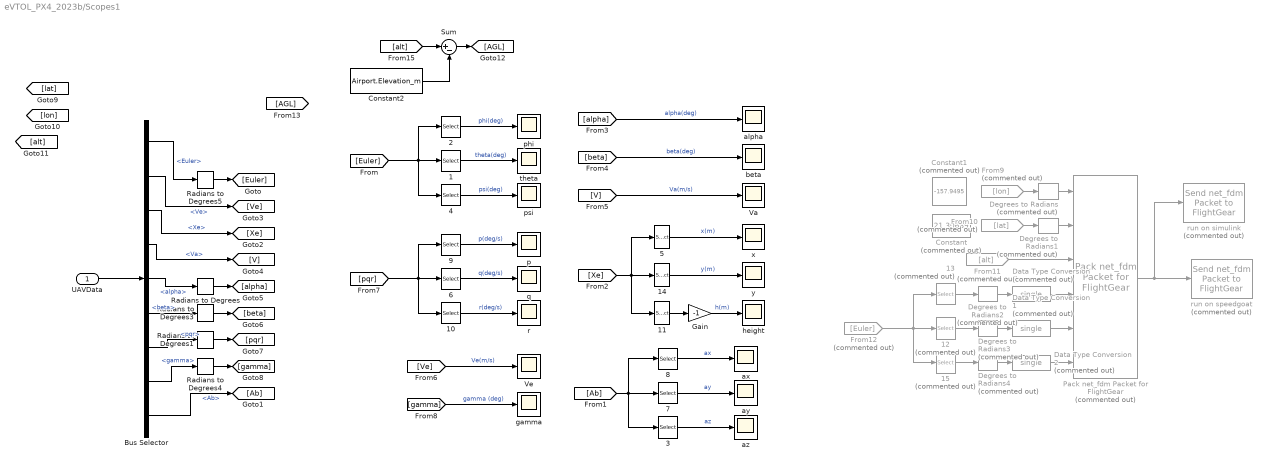
== system eVTOL_PX4_2023b/Scopes1 ==
  UAVData : Inport
  {1,6..7,14} (4 alike) : Selector  InputPortWidth=3  IndexOptions=Index vector (dialog)  Indices=2  OutputSizes=1
  {3..4,10..11} (4 alike) : Selector  InputPortWidth=3  IndexOptions=Index vector (dialog)  Indices=3  OutputSizes=1
  12 : Selector  Commented=on  InputPortWidth=3  IndexOptions=Index vector (dialog)  Indices=2  OutputSizes=1
  13 : Selector  Commented=on  InputPortWidth=3  IndexOptions=Index vector (dialog)  Indices=1  OutputSizes=1
  15 : Selector  Commented=on  InputPortWidth=3  IndexOptions=Index vector (dialog)  Indices=3  OutputSizes=1
  {2,5,8..9} (4 alike) : Selector  InputPortWidth=3  IndexOptions=Index vector (dialog)  Indices=1  OutputSizes=1
  Bus Selector : BusSelector  OutputSignals=Euler,Ve,Xe,Va,alpha,beta,pqr,gamma,Ab
  Constant : Constant  Commented=on  Value=21.30689
  Constant1 : Constant  Commented=on  Value=-157.9495
  Constant2 : Constant  Value=Airport.Elevation_m
  Data Type Conversion : DataTypeConversion  Commented=on  OutDataTypeStr=single  SaturateOnIntegerOverflow=off  RndMeth=Floor
  Data Type Conversion1 : DataTypeConversion  Commented=on  OutDataTypeStr=single  SaturateOnIntegerOverflow=off  RndMeth=Floor
  Data Type Conversion2 : DataTypeConversion  Commented=on  OutDataTypeStr=single  SaturateOnIntegerOverflow=off  RndMeth=Floor
  Degrees to Radians{,1..4} (5 alike) : simulink_extras/Transformations/Degrees to Radians  Commented=on
  From10 : From  Commented=on  GotoTag=lat
  From11 : From  Commented=on  GotoTag=alt
  From12 : From  Commented=on  GotoTag=Euler
  From9 : From  Commented=on  GotoTag=lon
  Gain : Gain  Gain=-1
  Pack net_fdm Packet for FlightGear : aerolibfltsims/Pack net_fdm Packet for FlightGear  Commented=on  FlightGearVersion=v2019.1  ShowPositionAttitudeInputs=on  ShowVelocityAccelerationInputs=off  ShowControlSurfacePositionInputs=off  ShowEngineFuelInputs=off  ShowLandingGearInputs=off  ShowEnvironmentInputs=off  SampleTime=-1  packetVersion=24
  Radians to Degrees{,1,3..5} (5 alike) : simulink_extras/Transformations/Radians to Degrees
  Sum : Sum  Inputs=|+-
  Va : Scope
  Ve : Scope
  alpha : Scope
  ax : Scope
  ay : Scope
  az : Scope
  beta : Scope
  gamma : Scope
  height : Scope
  p : Scope
  phi : Scope
  psi : Scope
  q : Scope
  r : Scope
  run on simulink : aerolibfltsims/Send net_fdm Packet to FlightGear  Commented=on  DestinationIpAddress=127.0.0.1  DestinationPort=5502  LocalIpPort=-1  varLen=off  SampleTime=0.01
  run on speedgoat : aerolibfltsims/Send net_fdm Packet to FlightGear  Commented=on  DestinationIpAddress=192.168.7.2  DestinationPort=5502  LocalIpPort=-1  varLen=off  SampleTime=-1
  theta : Scope
  x : Scope
  y : Scope
  wires:
  Radians to Degrees5/1 -> [Euler]
  UAVData/1 -> Bus Selector/1
  1/1 -> theta/1  "theta(deg)"
  Bus Selector/3 -> [Xe]  "<Xe>"
  2/1 -> phi/1  "phi(deg)"
  4/1 -> psi/1  "psi(deg)"
  Bus Selector/5 -> Radians to Degrees/1  "<alpha>"
  [Euler] -> 1/1, 2/1, 4/1
  Bus Selector/1 -> Radians to Degrees5/1  "<Euler>"
  [Xe] -> 5/1, 14/1, 11/1
  Bus Selector/2 -> [Ve]  "<Ve>"
  Bus Selector/4 -> [V]  "<Va>"
  Radians to Degrees/1 -> [alpha]
  Bus Selector/6 -> Radians to Degrees3/1  "<beta>"
  Radians to Degrees3/1 -> [beta]
  [beta] -> beta/1  "beta(deg)"
  [alpha] -> alpha/1  "alpha(deg)"
  [Ve] -> Ve/1  "Ve(m/s)"
  Bus Selector/7 -> Radians to Degrees1/1  "<pqr>"
  6/1 -> q/1  "q(deg/s)"
  9/1 -> p/1  "p(deg/s)"
  10/1 -> r/1  "r(deg/s)"
  [pqr] -> 10/1, 9/1, 6/1
  Radians to Degrees1/1 -> [pqr]
  11/1 -> Gain/1
  Gain/1 -> height/1  "h(m)"
  5/1 -> x/1  "x(m)"
  Bus Selector/8 -> Radians to Degrees4/1  "<gamma>"
  Radians to Degrees4/1 -> [gamma]
  [gamma] -> gamma/1  "gamma (deg)"
  14/1 -> y/1  "y(m)"
  [V] -> Va/1  "Va(m/s)"
  Bus Selector/9 -> [Ab]  "<Ab>"
  [Ab] -> 8/1, 7/1, 3/1
  3/1 -> az/1  "az"
  8/1 -> ax/1  "ax"
  7/1 -> ay/1  "ay"
  ? -> [lat]  "<lat_deg>"
  ? -> [lon]  "<lon_deg>"
  ? -> [alt]  "<AMSL>"
  Pack net_fdm Packet for FlightGear/1 -> run on simulink/1, run on speedgoat/1
  Degrees to Radians1/1 -> Pack net_fdm Packet for FlightGear/2
  Data Type Conversion/1 -> Pack net_fdm Packet for FlightGear/4
  Degrees to Radians/1 -> Pack net_fdm Packet for FlightGear/1
  12/1 -> Degrees to Radians3/1
  Data Type Conversion1/1 -> Pack net_fdm Packet for FlightGear/5
  13/1 -> Degrees to Radians2/1
  15/1 -> Degrees to Radians4/1
  Data Type Conversion2/1 -> Pack net_fdm Packet for FlightGear/6
  From11/1 -> Pack net_fdm Packet for FlightGear/3
  Degrees to Radians2/1 -> Data Type Conversion/1
  Degrees to Radians3/1 -> Data Type Conversion1/1
  Degrees to Radians4/1 -> Data Type Conversion2/1
  From9/1 -> Degrees to Radians/1
  From10/1 -> Degrees to Radians1/1
  From12/1 -> 15/1, 13/1, 12/1
  Constant2/1 -> Sum/2
  Sum/1 -> [AGL]
  [alt] -> Sum/1

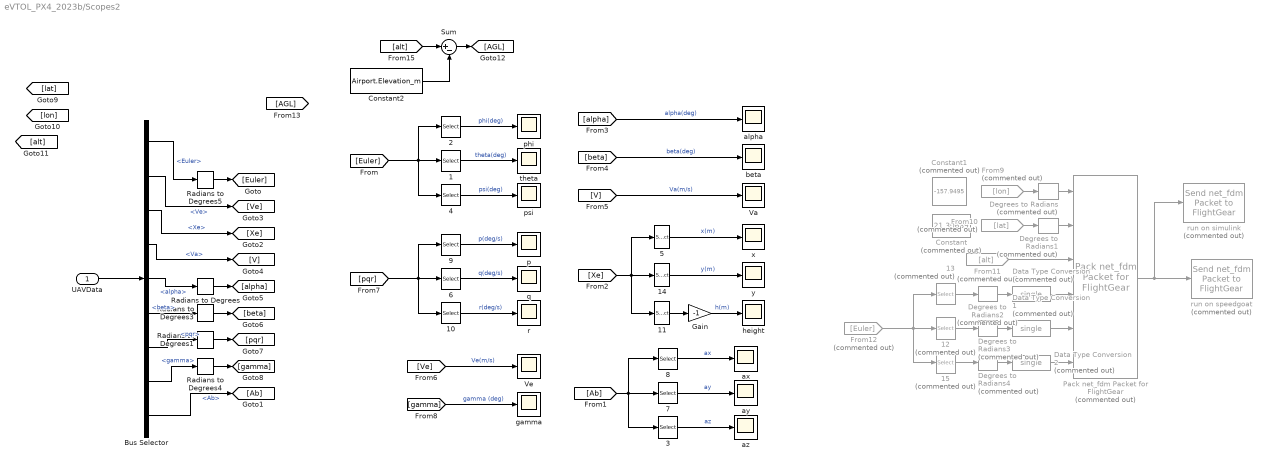
== system eVTOL_PX4_2023b/Scopes2 ==
  UAVData : Inport
  {1,6..7,14} (4 alike) : Selector  InputPortWidth=3  IndexOptions=Index vector (dialog)  Indices=2  OutputSizes=1
  {3..4,10..11} (4 alike) : Selector  InputPortWidth=3  IndexOptions=Index vector (dialog)  Indices=3  OutputSizes=1
  12 : Selector  Commented=on  InputPortWidth=3  IndexOptions=Index vector (dialog)  Indices=2  OutputSizes=1
  13 : Selector  Commented=on  InputPortWidth=3  IndexOptions=Index vector (dialog)  Indices=1  OutputSizes=1
  15 : Selector  Commented=on  InputPortWidth=3  IndexOptions=Index vector (dialog)  Indices=3  OutputSizes=1
  {2,5,8..9} (4 alike) : Selector  InputPortWidth=3  IndexOptions=Index vector (dialog)  Indices=1  OutputSizes=1
  Bus Selector : BusSelector  OutputSignals=Euler,Ve,Xe,Va,alpha,beta,pqr,gamma,Ab
  Constant : Constant  Commented=on  Value=21.30689
  Constant1 : Constant  Commented=on  Value=-157.9495
  Constant2 : Constant  Value=Airport.Elevation_m
  Data Type Conversion : DataTypeConversion  Commented=on  OutDataTypeStr=single  SaturateOnIntegerOverflow=off  RndMeth=Floor
  Data Type Conversion1 : DataTypeConversion  Commented=on  OutDataTypeStr=single  SaturateOnIntegerOverflow=off  RndMeth=Floor
  Data Type Conversion2 : DataTypeConversion  Commented=on  OutDataTypeStr=single  SaturateOnIntegerOverflow=off  RndMeth=Floor
  Degrees to Radians{,1..4} (5 alike) : simulink_extras/Transformations/Degrees to Radians  Commented=on
  From10 : From  Commented=on  GotoTag=lat
  From11 : From  Commented=on  GotoTag=alt
  From12 : From  Commented=on  GotoTag=Euler
  From9 : From  Commented=on  GotoTag=lon
  Gain : Gain  Gain=-1
  Pack net_fdm Packet for FlightGear : aerolibfltsims/Pack net_fdm Packet for FlightGear  Commented=on  FlightGearVersion=v2019.1  ShowPositionAttitudeInputs=on  ShowVelocityAccelerationInputs=off  ShowControlSurfacePositionInputs=off  ShowEngineFuelInputs=off  ShowLandingGearInputs=off  ShowEnvironmentInputs=off  SampleTime=-1  packetVersion=24
  Radians to Degrees{,1,3..5} (5 alike) : simulink_extras/Transformations/Radians to Degrees
  Sum : Sum  Inputs=|+-
  Va : Scope
  Ve : Scope
  alpha : Scope
  ax : Scope
  ay : Scope
  az : Scope
  beta : Scope
  gamma : Scope
  height : Scope
  p : Scope
  phi : Scope
  psi : Scope
  q : Scope
  r : Scope
  run on simulink : aerolibfltsims/Send net_fdm Packet to FlightGear  Commented=on  DestinationIpAddress=127.0.0.1  DestinationPort=5502  LocalIpPort=-1  varLen=off  SampleTime=0.01
  run on speedgoat : aerolibfltsims/Send net_fdm Packet to FlightGear  Commented=on  DestinationIpAddress=192.168.7.2  DestinationPort=5502  LocalIpPort=-1  varLen=off  SampleTime=-1
  theta : Scope
  x : Scope
  y : Scope
  wires:
  Radians to Degrees5/1 -> [Euler]
  UAVData/1 -> Bus Selector/1
  1/1 -> theta/1  "theta(deg)"
  Bus Selector/3 -> [Xe]  "<Xe>"
  2/1 -> phi/1  "phi(deg)"
  4/1 -> psi/1  "psi(deg)"
  Bus Selector/5 -> Radians to Degrees/1  "<alpha>"
  [Euler] -> 1/1, 2/1, 4/1
  Bus Selector/1 -> Radians to Degrees5/1  "<Euler>"
  [Xe] -> 5/1, 14/1, 11/1
  Bus Selector/2 -> [Ve]  "<Ve>"
  Bus Selector/4 -> [V]  "<Va>"
  Radians to Degrees/1 -> [alpha]
  Bus Selector/6 -> Radians to Degrees3/1  "<beta>"
  Radians to Degrees3/1 -> [beta]
  [beta] -> beta/1  "beta(deg)"
  [alpha] -> alpha/1  "alpha(deg)"
  [Ve] -> Ve/1  "Ve(m/s)"
  Bus Selector/7 -> Radians to Degrees1/1  "<pqr>"
  6/1 -> q/1  "q(deg/s)"
  9/1 -> p/1  "p(deg/s)"
  10/1 -> r/1  "r(deg/s)"
  [pqr] -> 10/1, 9/1, 6/1
  Radians to Degrees1/1 -> [pqr]
  11/1 -> Gain/1
  Gain/1 -> height/1  "h(m)"
  5/1 -> x/1  "x(m)"
  Bus Selector/8 -> Radians to Degrees4/1  "<gamma>"
  Radians to Degrees4/1 -> [gamma]
  [gamma] -> gamma/1  "gamma (deg)"
  14/1 -> y/1  "y(m)"
  [V] -> Va/1  "Va(m/s)"
  Bus Selector/9 -> [Ab]  "<Ab>"
  [Ab] -> 8/1, 7/1, 3/1
  3/1 -> az/1  "az"
  8/1 -> ax/1  "ax"
  7/1 -> ay/1  "ay"
  ? -> [lat]  "<lat_deg>"
  ? -> [lon]  "<lon_deg>"
  ? -> [alt]  "<AMSL>"
  Pack net_fdm Packet for FlightGear/1 -> run on simulink/1, run on speedgoat/1
  Degrees to Radians1/1 -> Pack net_fdm Packet for FlightGear/2
  Data Type Conversion/1 -> Pack net_fdm Packet for FlightGear/4
  Degrees to Radians/1 -> Pack net_fdm Packet for FlightGear/1
  12/1 -> Degrees to Radians3/1
  Data Type Conversion1/1 -> Pack net_fdm Packet for FlightGear/5
  13/1 -> Degrees to Radians2/1
  15/1 -> Degrees to Radians4/1
  Data Type Conversion2/1 -> Pack net_fdm Packet for FlightGear/6
  From11/1 -> Pack net_fdm Packet for FlightGear/3
  Degrees to Radians2/1 -> Data Type Conversion/1
  Degrees to Radians3/1 -> Data Type Conversion1/1
  Degrees to Radians4/1 -> Data Type Conversion2/1
  From9/1 -> Degrees to Radians/1
  From10/1 -> Degrees to Radians1/1
  From12/1 -> 15/1, 13/1, 12/1
  Constant2/1 -> Sum/2
  Sum/1 -> [AGL]
  [alt] -> Sum/1

== system eVTOL_PX4_2023b/Sensors ==
  UAVData : Inport
  Bus Creator : BusCreator  Inputs=24
  Bus Selector : BusSelector  OutputSignals=Ve,Xe,Euler,DCM_be,Vb,pqr,pqr_dot,Ab,alpha,alphaDot,beta,Va,pqrWind,mach,Q,gamma,chi,Po,To,g,mass
  Constant : Constant  Value=Airport.Elevation_m
  Divide : Product  Inputs=**  Multiplication=Matrix(*)
  Flat Earth to LLA : aerolibtransform2/Flat Earth to LLA  units=Metric (MKS)  ptype=Earth (WGS84)  F=1/298.257223563  R=6378137  refPosPort=off  LL0=InitData.LLA(1:2)*R2D  psi=0
  Gain : Gain  Gain=-1
  Mux : Mux  Inputs=2
  Scope : Scope
  Scope1 : Scope
  Scope2 : Scope
  Selector : Selector  InputPortWidth=3  IndexOptions=Index vector (dialog)  Indices=3  OutputSizes=1
  Selector1 : Selector  InputPortWidth=3  IndexOptions=Index vector (dialog)  Indices=3  OutputSizes=1
  Transpose : Math  Operator=transpose
  SensorData : Outport
  wires:
  Constant/1 -> Flat Earth to LLA/2
  Flat Earth to LLA/1 -> Mux/1
  Flat Earth to LLA/2 -> [AGL]  "AGL"
  UAVData/1 -> Bus Selector/1
  Bus Selector/2 -> [Xe]  "<Xe>"
  [Xe] -> Selector/1, Flat Earth to LLA/1
  Bus Selector/8 -> Scope/1, [Ab]  "<Ab>"
  Bus Selector/4 -> [DCM_be]  "<DCM_be>"
  [DCM_be] -> Transpose/1
  [Ab] -> Divide/2
  Selector/1 -> Gain/1
  Gain/1 -> Mux/2
  Mux/1 -> [LLA_deg]  "LLA_deg"
  Bus Selector/1 -> [Ve]  "<Ve>"
  Bus Selector/3 -> [Euler]  "<Euler>"
  Bus Selector/5 -> [Vb]  "<Vb>"
  Bus Selector/6 -> [pqr]  "<pqr>"
  Bus Selector/7 -> [pqr_dot]  "<pqr_dot>"
  Bus Selector/9 -> [alpha]  "<alpha>"
  Bus Selector/10 -> [alpha_dot]  "<alphaDot>"
  Bus Selector/11 -> [beta]  "<beta>"
  Bus Selector/12 -> [Va]  "<Va>"
  Bus Selector/13 -> [pwrWind]  "<pqrWind>"
  Bus Selector/14 -> [mach]  "<mach>"
  Bus Selector/15 -> [Q]  "<Q>"
  Bus Selector/16 -> [gamma]  "<gamma>"
  Bus Selector/17 -> [chi]  "<chi>"
  Bus Selector/18 -> [Po]  "<Po>"
  Bus Selector/19 -> [To]  "<To>"
  Bus Selector/20 -> [g]  "<g>"
  Bus Selector/21 -> [mass]  "<mass>"
  Transpose/1 -> Divide/1
  Divide/1 -> [Ae]  "Ae"
  [Xe] -> Bus Creator/3
  [Ve] -> Bus Creator/4
  [Ae] -> Bus Creator/5
  [Vb] -> Bus Creator/6
  [Ab] -> Bus Creator/7
  [DCM_be] -> Bus Creator/8
  [Euler] -> Bus Creator/9
  [AGL] -> Bus Creator/2
  [pqr] -> Bus Creator/10
  [pqr_dot] -> Bus Creator/11
  [alpha] -> Bus Creator/13
  [beta] -> Bus Creator/14
  [alpha_dot] -> Bus Creator/15
  [Va] -> Scope1/1, Bus Creator/16
  [mach] -> Bus Creator/17
  [pwrWind] -> Bus Creator/12
  [chi] -> Bus Creator/18
  [gamma] -> Bus Creator/19
  [Q] -> Bus Creator/20
  [Po] -> Bus Creator/21
  [To] -> Bus Creator/22
  [g] -> Bus Creator/23
  [mass] -> Bus Creator/24
  Bus Creator/1 -> SensorData/1
  [LLA_deg] -> Selector1/1, Bus Creator/1
  Selector1/1 -> Scope2/1  "h"

== system eVTOL_PX4_2023b/Subsystem1 ==
  ActData : Inport
  SW : Inport  Port=2
  Bus Selector : BusSelector  OutputSignals=Act_surface,Act_T
  Energy & Power : Subsystem  Commented=on
  Energy & Power1 : Subsystem
  Environment : Subsystem  Commented=on  AncestorBlock=asbhl20env/Environment  TreatAsAtomicUnit=on
      settings: LibrarySourceBlock=asbhl20env/Environment
  Environment1 : Subsystem  AncestorBlock=asbhl20env/Environment  TreatAsAtomicUnit=on
      settings: LibrarySourceBlock=asbhl20env/Environment
  airframe : Subsystem  Commented=on
  airframe1 : Subsystem
  UAVData : Outport
  wires:
  airframe/1(UAVData) -> Energy & Power/2(UAVData), Environment/1(plane)
  Energy & Power/1(PropData) -> airframe/2(prop)
  Environment/1(Envm) -> Energy & Power/1(EnvData), airframe/1(EnvmData)
  ActData/1 -> Bus Selector/1
  Energy & Power1/1(PropData) -> airframe1/2(prop)
  Environment1/1(Envm) -> Energy & Power1/1(EnvData), airframe1/1(EnvmData)
  airframe1/1(UAVData) -> UAVData/1, Environment1/1(plane), Energy & Power1/2(UAVData)
  Bus Selector/2 -> Energy & Power1/3(Act_T)  "<Act_T>"
  Bus Selector/1 -> airframe1/3(Act_surface)  "<Act_surface>"
  SW/1 -> airframe1/4(SW)

== system eVTOL_PX4_2023b/Subsystem2 ==
  ActData : Inport
  SW : Inport  Port=2
  Bus Selector : BusSelector  OutputSignals=Act_surface,Act_T
  Energy & Power : Subsystem
  Environment : Subsystem  AncestorBlock=asbhl20env/Environment  TreatAsAtomicUnit=on
      settings: LibrarySourceBlock=asbhl20env/Environment
  airframe : Subsystem
  UAVData : Outport
  wires:
  airframe/1(UAVData) -> UAVData/1, Energy & Power/2(UAVData), Environment/1(plane)
  Energy & Power/1(PropData) -> airframe/2(prop)
  SW/1 -> airframe/4(SW)
  Environment/1(Envm) -> Energy & Power/1(EnvData), airframe/1(EnvmData)
  Bus Selector/2 -> Energy & Power/3(Act_T)  "<Act_T>"
  ActData/1 -> Bus Selector/1
  Bus Selector/1 -> airframe/3(Act_surface)  "<Act_surface>"

== system eVTOL_PX4_2023b/UAV ==
  ActData : Inport
  SW : Inport  Port=2
  WindSpeed : Inport  Port=3
  Energy & Power : Subsystem
  Environment : Subsystem  AncestorBlock=asbhl20env/Environment  TreatAsAtomicUnit=on
  airframe : Subsystem
  UAVData : Outport
  wires:
  Environment/1(Envm) -> airframe/1(EnvmData)
  airframe/1(UAVData) -> UAVData/1, Energy & Power/1(UAVData), Environment/1(plane)
  ActData/1 -> Energy & Power/2(ActData), airframe/3(ActData)
  Energy & Power/1(PropData) -> airframe/2(PropData)
  SW/1 -> airframe/4(SW)
  WindSpeed/1 -> Environment/2(WindSpeed)

== system eVTOL_PX4_2023b/hil_state_quaternion_pack1 ==
  time_s : Inport
  DCM_be : Inport  Port=2
  body_rate : Inport  Port=3
  latlon_deg : Inport  Port=4
  amsl : Inport  Port=5
  Ve : Inport  Port=6
  ab : Inport  Port=7
  EAS : Inport  Port=8
  TAS : Inport  Port=9
  Bus Creator : BusCreator  Inputs=5  OutDataTypeStr=Bus: SL_Bus_MAVLink_HIL_STATE_QUATERNION_Packet  NonVirtualBus=on
  Bus Selector : BusSelector  OutputSignals=MsgID,SystemID,ComponentID,Sequence
  MAVLink Blank Message2 : uavmavlinklib/MAVLink Blank Message  dialectSource=Select from standard MAVLink dialects  dialect=common.xml  dialectCustom=common.xml  version=2  messageType=HIL_STATE_QUATERNION  SystemID=SYS_ID  ComponentID=COMP_ID  SampleTime=SAMPLE_TIME
  MAVLink Serializer2 : uavmavlinklib/MAVLink Serializer  dialectSource=Select from standard MAVLink dialects  dialect=common.xml  dialectCustom=common.xml  version=2  messageType=HIL_STATE_QUATERNION
  Signal Conversion : SignalConversion  ConversionOutput=Nonvirtual bus  OverrideOpt=off
  Terminator2 : Terminator
  payload_hil_state_quaternion : Subsystem
  Data to px4 : Outport
  wires:
  latlon_deg/1 -> payload_hil_state_quaternion/4(latlon_deg)
  MAVLink Serializer2/2 -> Terminator2/1
  MAVLink Serializer2/1 -> Data to px4/1  "status"
  MAVLink Blank Message2/1 -> Bus Selector/1
  payload_hil_state_quaternion/1(Payload) -> Bus Creator/5
  Bus Selector/3 -> Bus Creator/3  "<ComponentID>"
  Bus Selector/4 -> Bus Creator/4  "<Sequence>"
  Bus Selector/2 -> Bus Creator/2  "<SystemID>"
  Bus Selector/1 -> Bus Creator/1  "<MsgID>"
  time_s/1 -> payload_hil_state_quaternion/1(time_s)
  body_rate/1 -> payload_hil_state_quaternion/3(body_rate)
  amsl/1 -> payload_hil_state_quaternion/5(amsl)
  DCM_be/1 -> payload_hil_state_quaternion/2(DCM_be)
  Ve/1 -> payload_hil_state_quaternion/6(Ve)
  TAS/1 -> payload_hil_state_quaternion/9(TAS)
  ab/1 -> payload_hil_state_quaternion/7(ab)
  EAS/1 -> payload_hil_state_quaternion/8(EAS)
  Bus Creator/1 -> Signal Conversion/1
  Signal Conversion/1 -> MAVLink Serializer2/1

== system eVTOL_PX4_2023b/FCS/FCS CMD ==
  note: FlightMod
      | 1-Ready
      | 2-TakeOff
      | 3-PullUp
      | 4-Climb
      | 5-Cruise, 5.1-circle, 5.2-line
      | 6-Return
      | 7-Approach
      | 8-Flare
      | 9-TouchDown
      | 10-Taxi
      | 11-GoAround
      | 12-Parachute
  note: LonMod:
      | 1-theta hold
      | 2-height hold
      | 3-gamma control
      | 4-landing flare control
      | 5-TakeOff
  note: LatMod:
      | 1-phi hold
      | 2-lateral deviation control
      | 3-taxi y control
      | 4-
      | 5-taxi y control
  note: VMod:
      | 1-cruise throt
      | 2-max throt
      | 3-min throt
      | 4-TECS
      | 5-Flare dt Fade
  SensorData : Inport
  Land_SW : Inport  Port=2
  Bus Creator1 : BusCreator  Inputs=14
  Bus Selector : BusSelector  OutputSignals=Xe,Va,Euler
  Clock : Clock
  Divide : Product  Inputs=*/
  Divide1 : Product  Inputs=**
  Gain : Gain  Gain=-1
  Ground : Ground
  ISA Atmosphere Model : aerolibatmos2/ISA Atmosphere Model  useExtended=off  action=Warning  custom=off  viscosityOut=off  g=9.80665  gamma=1.4  R=287.0531  L=0.0065  h_trop=11000  h_strat=20000  rho0=1.225  P0=101325  T0=288.15  h0=0
  Mode Generator : Stateflow chart  TreatAsAtomicUnit=on
  Rate Limiter : RateLimiter  RisingSlewLimit=10  FallingSlewLimit=-5  SampleTimeMode=inherited
  Scope : Scope
  Selector : Selector  InputPortWidth=3  IndexOptions=Index vector (dialog)  Indices=[1]  OutputSizes=1
  Selector1 : Selector  InputPortWidth=3  IndexOptions=Index vector (dialog)  Indices=2  OutputSizes=1
  Selector2 : Selector  InputPortWidth=3  IndexOptions=Index vector (dialog)  Indices=3  OutputSizes=1
  Selector3 : Selector  InputPortWidth=3  IndexOptions=Index vector (dialog)  Indices=3  OutputSizes=1
  Sqrt : Sqrt
  Terminator : Terminator
  Terminator1 : Terminator
  Terminator2 : Terminator
  hground_value : Constant  Value=Airport.Elevation_m  OutDataTypeStr=double
  phic1 : Constant  Value=1.225
  FCSCMD : Outport  VectorParamsAs1DForOutWhenUnconnected=off
  tag scope: icmd=global
  wires:
  [V] -> Mode Generator/3(V)
  [H] -> Mode Generator/1(H)
  Clock/1 -> Mode Generator/5(time)
  Mode Generator/12(L1mod) -> Bus Creator1/12  "L1Mod"
  Mode Generator/6(Vmod) -> Bus Creator1/6  "VMod"
  Mode Generator/2(Lonmod) -> Bus Creator1/2  "LonMod"
  Mode Generator/3(thetac) -> Bus Creator1/3  "thetac"
  Mode Generator/7(Vc) -> Divide1/1, Bus Creator1/7  "Vc_EAS"
  Mode Generator/8(Latmod) -> Bus Creator1/8  "LatMod"
  Mode Generator/4(gammac) -> Bus Creator1/4  "gammac"
  Mode Generator/9(phic) -> Bus Creator1/9  "phic"
  Mode Generator/11(yc) -> Bus Creator1/11  "yc"
  Mode Generator/10(chic) -> Bus Creator1/10  "chic"
  [x] -> Mode Generator/2(x)
  SensorData/1 -> Bus Selector/1
  Bus Selector/1 -> Selector/1, Selector1/1, Selector3/1  "<Xe>"
  Selector3/1 -> Gain/1
  Selector/1 -> [x]
  Gain/1 -> [H]
  Bus Selector/2 -> [V]  "<Va>"
  Ground/1 -> Mode Generator/6(psi0)
  Bus Selector/3 -> Selector2/1  "<Euler>"
  Selector2/1 -> [psi]
  Selector1/1 -> [y]
  hground_value/1 -> Mode Generator/4(h_runway)
  Mode Generator/1(FlightMod) -> Scope/1, Bus Creator1/1  "FlightMod"
  Bus Creator1/1 -> FCSCMD/1  "FCSCMD"
  [H] -> ISA Atmosphere Model/1
  ISA Atmosphere Model/4 -> Divide/2  "rho"
  phic1/1 -> Divide/1
  Divide/1 -> Sqrt/1
  Sqrt/1 -> Divide1/2
  Divide1/1 -> Bus Creator1/13  "Vc_TAS"
  ISA Atmosphere Model/1 -> Terminator/1
  ISA Atmosphere Model/2 -> Terminator1/1
  ISA Atmosphere Model/3 -> Terminator2/1
  Land_SW/1 -> Mode Generator/7(LAND_SW)
  Mode Generator/13(icmd) -> [icmd], Bus Creator1/14  "icmd"
  Mode Generator/5(hc) -> Rate Limiter/1  "Hc"
  Rate Limiter/1 -> Bus Creator1/5  "Hc"
